simulink model "AvionicStateFlow1"  (R2021a)
settings: Solver=FixedStepAuto  StartTime=0.0  StopTime=inf  FixedStep=0.01  RelTol=1e-3  EnableMultiTasking=on
libraries: bbblueCommlib x27, svdutilitieslib x10, simulink x5, bbblueBasicLib x4, bbblueSensorLib x2
settings Model: SimulationMode=external  ExtModeTrigDuration=100  Creator=SONG PC  LastModifiedBy=sokserey
settings SolverCC: PositivePriorityOrder=on  AutoInsertRateTranBlk=on
settings OptimizationCC: EnhancedBackFolding=on  PassReuseOutputArgsAs=Individual arguments  ZeroExternalMemoryAtStartup=off  ZeroInternalMemoryAtStartup=off  MaxStackSize=64  OptimizeBlockOrder=speed  DifferentSizesBufferReuse=on  OptimizationCustomize=off  EfficientTunableParamExpr=on
settings DebuggingCC: ParameterTunabilityLossMsg=error
settings HardwareCC: ProdBitPerPointer=32  ProdBitPerSizeT=32  ProdBitPerPtrDiffT=32  ProdLargestAtomicInteger=Long  ProdLargestAtomicFloat=Double  ProdWordSize=32  ProdHWDeviceType=ARM Compatible->ARM Cortex
settings SFSimCC: MATLABDynamicMemAlloc=off
settings RTWCC: SystemTargetFile=ert.tlc  HardwareBoard=BeagleBone Blue  TLCOptions="-aInlineSetEventsForThisBaseRateFcn=TLC_FALSE -aSuppressMultiTaskScheduler=TLC_FALSE  -aRateBasedStepFcn=0"  TemplateMakefile=ert_default_tmf  Toolchain=GNU GCC BeagleBone Blue
settings CodeAppCC: ForceParamTrailComments=on  IgnoreCustomStorageClasses=off  OperatorAnnotations=on  SimulinkDataObjDesc=on  SFDataObjDesc=on  InsertBlockDesc=on
settings ERTTargetCC: SupportContinuousTime=on  SupportVariableSizeSignals=on  ExtMode=on  ExtModeMexArgs='192.168.7.2' 0 17725

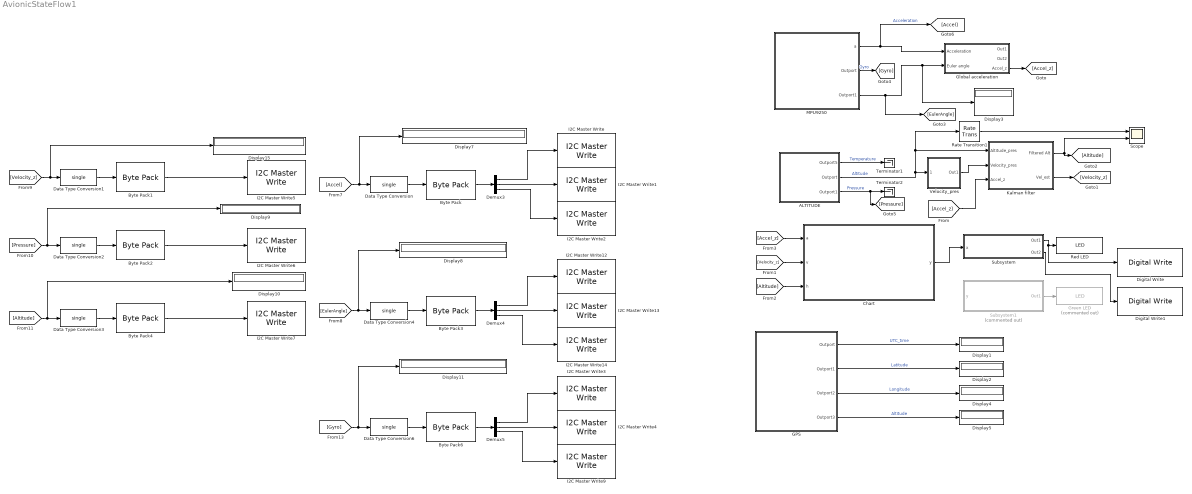
== system AvionicStateFlow1 ==
  "ALTITUDE " : Subsystem
  Byte Pack{,1..4,6} (6 alike) : svdutilitieslib/Byte Pack  maskPackedDataType=uint8  datatypes={'single'}  byteAlign=1  blockPlatform=arduinoert
      settings: SourceProductBaseCode=ARDUINO,ML_ARDUINO,ECCORTEXA,ECCORTEXR,SC_BEAGLEBONE_BLUE,EC_FREEDOM_BOARD,EC_FRDM_K64F,INTEL_BLOCKSET,MICROBIT,NUCLEO,PX4AUTOPILOTS,RASPPIIO,STMICRODIS,TIC2000,XILINX_BLOCKSET
  Chart : Stateflow chart  TreatAsAtomicUnit=on
  Data Type Conversion{,1..4,6} (6 alike) : DataTypeConversion  OutDataTypeStr=single
  Demux3 : Demux  Outputs=3
  Demux4 : Demux  Outputs=3
  Demux5 : Demux  Outputs=3
  Digital Write : bbblueBasicLib/Digital Write  GPIOSelect=GPIO1_25  Pin=49  Direction=output
      settings: SourceProductBaseCode=SC_BEAGLEBONE_BLUE
  Digital Write1 : bbblueBasicLib/Digital Write  GPIOSelect=GPIO3_2  Pin=49  Direction=output
      settings: SourceProductBaseCode=SC_BEAGLEBONE_BLUE
  Display{1..5,7..11,15} (11 alike) : Display
  GPS : Subsystem
  Global acceleration : Subsystem
  Green LED : bbblueBasicLib/LED  Commented=on  LED=Green
      settings: SourceProductBaseCode=SC_BEAGLEBONE_BLUE
  I2C Master Write{,1..7,9,12..14} (12 alike) : bbblueCommlib/I2C Master Write  I2CModule=1  Mode=Master  SlaveAddress=8  SlaveByteOrder=BigEndian  Direction=Transmitter  RegisterAddressMode=off  RegisterAddress=0  SlaveDataType=uint8  DataLength=1  NoAck=off  RepeatedStart=off  OutputStatus=off
      settings: SourceProductBaseCode=SC_BEAGLEBONE_BLUE
  Kalman filter : Subsystem
  MPU9250 : Subsystem
  Rate Transition1 : RateTransition
  Red LED : bbblueBasicLib/LED  LED=Red
      settings: SourceProductBaseCode=SC_BEAGLEBONE_BLUE
  Scope : Scope  NumInputPorts=2
  Subsystem : Subsystem
  Subsystem1 : Subsystem  Commented=on
  Terminator1 : Terminator
  Terminator2 : Terminator
  Velocity_pres : Subsystem
  wires:
  "ALTITUDE "/2(Outport) -> Velocity_pres/1(Altitude), Rate Transition1/1, Kalman filter/1(Altitude_pres)  "Altitude"
  "ALTITUDE "/3(Outport1) -> [Pressure], Terminator2/1  "Pressure"
  "ALTITUDE "/1(Outport5) -> Terminator1/1  "Temperature"
  Rate Transition1/1 -> Scope/1
  Subsystem/1(Out1) -> Digital Write/1, Red LED/1
  Subsystem1/1(Out1) -> Green LED/1
  MPU9250/1(a) -> [Accel], Global acceleration/1(Acceleration)  "Acceleration"
  Kalman filter/1(Filtered Alt) -> Scope/2, [Altitude]
  Kalman filter/2(Vel_est) -> [Velocity_z]
  Global acceleration/3(Accel_z) -> [Accel_z]
  [Accel_z] -> Kalman filter/3(Accel_z)
  [Accel_z] -> Chart/1(a)
  [Velocity_z] -> Chart/2(v)
  [Altitude] -> Chart/3(h)
  Velocity_pres/1(Out1) -> Kalman filter/2(Velocity_pres)
  Chart/1(y) -> Subsystem/1(x)
  Subsystem/2(Out2) -> Digital Write1/1
  Data Type Conversion6/1 -> Byte Pack6/1
  Byte Pack3/1 -> Demux4/1
  Demux5/1 -> I2C Master Write3/1
  Demux3/1 -> I2C Master Write/1
  Byte Pack2/1 -> I2C Master Write6/1
  [EulerAngle] -> Display8/1, Data Type Conversion4/1
  Byte Pack1/1 -> I2C Master Write5/1
  Data Type Conversion1/1 -> Byte Pack1/1
  Byte Pack6/1 -> Demux5/1
  Demux3/2 -> I2C Master Write1/1
  Byte Pack/1 -> Demux3/1
  Demux5/3 -> I2C Master Write9/1
  Demux4/3 -> I2C Master Write14/1
  Byte Pack4/1 -> I2C Master Write7/1
  [Altitude] -> Display10/1, Data Type Conversion3/1
  [Velocity_z] -> Display15/1, Data Type Conversion1/1
  Demux4/2 -> I2C Master Write13/1
  [Gyro] -> Display11/1, Data Type Conversion6/1
  Demux5/2 -> I2C Master Write4/1
  [Pressure] -> Display9/1, Data Type Conversion2/1
  [Accel] -> Display7/1, Data Type Conversion/1
  Demux4/1 -> I2C Master Write12/1
  Data Type Conversion3/1 -> Byte Pack4/1
  Data Type Conversion/1 -> Byte Pack/1
  Demux3/3 -> I2C Master Write2/1
  Data Type Conversion4/1 -> Byte Pack3/1
  Data Type Conversion2/1 -> Byte Pack2/1
  MPU9250/3(Outport1) -> [EulerAngle], Display3/1, Global acceleration/2(Euler angle)
  MPU9250/2(Outport) -> [Gyro]  "Gyro"
  GPS/2(Outport1) -> Display2/1  "Latitude"
  GPS/3(Outport2) -> Display4/1  "Longitude"
  GPS/4(Outport3) -> Display5/1  "Altitude"
  GPS/1(Outport) -> Display1/1  "UTC_time"

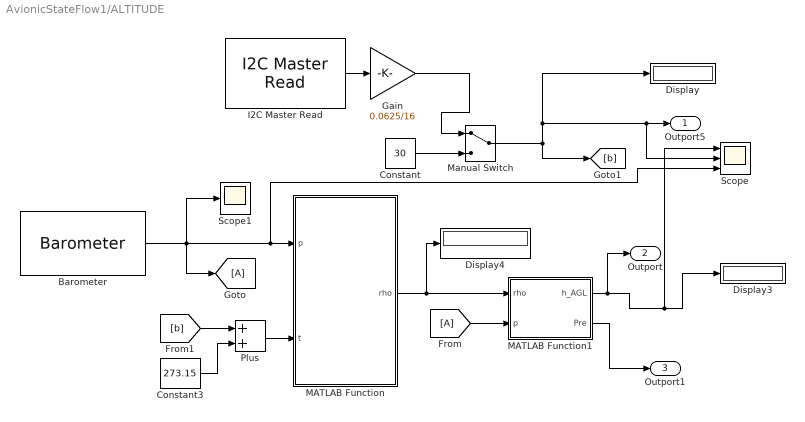
== system AvionicStateFlow1/ALTITUDE  ==
  Barometer : bbblueSensorLib/Barometer  OSRSelection=16  IIRFilterCoeff=16  SampleTime=0.01
      settings: SourceProductBaseCode=SC_BEAGLEBONE_BLUE
  Constant : Constant  Value=30
  Constant3 : Constant  Value=273.15
  Display : Display
  Display3 : Display
  Display4 : Display
  Gain : Gain  Gain=0.0625/16  OutDataTypeStr=single
  I2C Master Read : bbblueCommlib/I2C Master Read  I2CModule=1  Mode=Master  SlaveAddress=hex2dec('48')  SlaveByteOrder=BigEndian  Direction=Receiver  RegisterAddressMode=off  RegisterAddress=0  SlaveDataType=int16  DataLength=1  NoAck=off  RepeatedStart=off  OutputStatus=off  SampleTime=0.01
      settings: SourceProductBaseCode=SC_BEAGLEBONE_BLUE
  MATLAB Function : MATLAB Function  TreatAsAtomicUnit=on
  MATLAB Function1 : MATLAB Function  TreatAsAtomicUnit=on
  Manual Switch : ManualSwitch
  Plus : Sum
  Scope : Scope  NumInputPorts=3
  Scope1 : Scope
  Outport5 : Outport
  Outport : Outport  Port=2
  Outport1 : Outport  Port=3
  wires:
  I2C Master Read/1 -> Gain/1
  Plus/1 -> MATLAB Function/2(t)
  Barometer/1 -> Scope1/1, [A], Scope/3, MATLAB Function/1(p)
  Gain/1 -> Manual Switch/1
  MATLAB Function/1(rho) -> Display4/1, MATLAB Function1/1(rho)
  Constant3/1 -> Plus/2
  [A] -> MATLAB Function1/2(p)
  [b] -> Plus/1
  MATLAB Function1/1(h_AGL) -> Outport/1, Display3/1, Scope/1
  MATLAB Function1/2(Pre) -> Outport1/1
  Constant/1 -> Manual Switch/2
  Manual Switch/1 -> [b], Display/1, Scope/2, Outport5/1

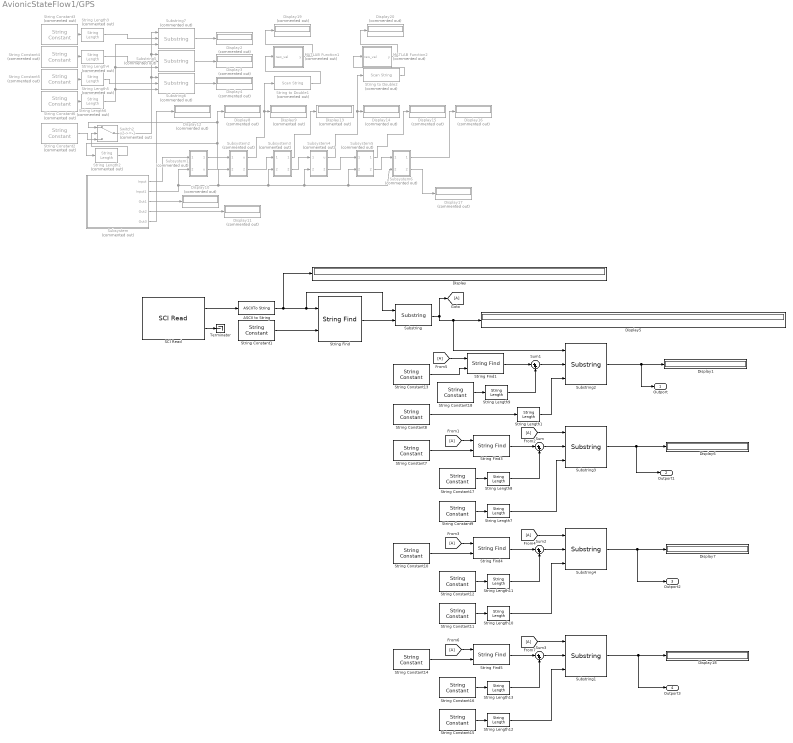
== system AvionicStateFlow1/GPS ==
  ASCII to String : ASCIIToString
  Display{,1,5..7,18} (6 alike) : Display
  Display{2..4,8..17,19..20} (15 alike) : Display  Commented=on
  MATLAB Function1 : MATLAB Function  Commented=on  TreatAsAtomicUnit=on
  MATLAB Function2 : MATLAB Function  Commented=on  TreatAsAtomicUnit=on
  SCI Read : bbblueCommlib/SCI Read  SCIModule=/dev/ttyO2  BaudrateOptions=9600  Parity=None  StopbitOptions=1  Baudrate=uint32(9600)  StopBits=1  HardwareFlowControl=None  ByteOrder=LittleEndian  DataType=uint8  DataLength=150  OutputStatus=on  SampleTime=0.1
      settings: SourceProductBaseCode=SC_BEAGLEBONE_BLUE
  String Constant1 : StringConstant  String="\"$GPGGA\""
  String Constant{7,10,13..14} (4 alike) : StringConstant  String="\",\""
  String Constant11 : StringConstant  String="\"hhhhhhhhhh\""
  String Constant12 : StringConstant  String="\"123456789101111111111111\""
  String Constant15 : StringConstant  String="\"hhhh\""
  String Constant16 : StringConstant  String="\"123456789101111111111111111111111111111111111111\""
  String Constant17 : StringConstant  String="\"12345678910\""
  String Constant18 : StringConstant  String="\"1\""
  String Constant2 : StringConstant  Commented=on  String="\"000000\""
  String Constant3 : StringConstant  Commented=on  String="\"0\""
  String Constant4 : StringConstant  Commented=on  String="\"000\""
  String Constant5 : StringConstant  Commented=on  String="\"00000\""
  String Constant6 : StringConstant  Commented=on  String="\"00\""
  String Constant8 : StringConstant  String="\"hhhhhh\""
  String Constant9 : StringConstant  String="\"hhhhhhhhhh\""
  String Find{,1,3..5} (5 alike) : StringFind
  String Length{1,7,10,12} (4 alike) : StringLength
  String Length{8..9,11,13} (4 alike) : StringLength  OutDataTypeStr=int32
  String Length{2..6} (5 alike) : StringLength  Commented=on
  String to Double1 : ScanString  Commented=on  Format="\"%lf\""
  String to Double2 : ScanString  Commented=on  Format="\"%lf\""
  Substring : Substring  StringFromIdxToEnd=on
  Substring{1..4} (4 alike) : Substring
  Substring5 : Substring  Commented=on
  Substring6 : Substring  Commented=on
  Substring7 : Substring  Commented=on
  Subsystem : Subsystem  Commented=on
  Subsystem1 : Subsystem  Commented=on
  Subsystem2 : Subsystem  Commented=on
  Subsystem3 : Subsystem  Commented=on
  Subsystem4 : Subsystem  Commented=on
  Subsystem5 : Subsystem  Commented=on
  Subsystem6 : Subsystem  Commented=on
  Sum{,1..3} (4 alike) : Sum  Inputs=|++
  Switch2 : Switch  Commented=on  Threshold=1
  Terminator : Terminator
  Outport : Outport
  Outport1 : Outport  Port=2
  Outport2 : Outport  Port=3
  Outport3 : Outport  Port=4
  wires:
  Switch2/1 -> Substring6/1, Substring5/1, Substring7/1
  String Length6/1 -> Substring6/3, Substring7/3, Substring5/3
  String Length4/1 -> Substring5/2
  String Length3/1 -> Substring7/2
  Subsystem5/1(Out1) -> Display15/1
  Subsystem/5(Out3) -> Display12/1
  Substring6/1 -> Display4/1
  String Constant5/1 -> String Length5/1
  String Constant4/1 -> String Length4/1
  String Length2/1 -> Switch2/2
  String Constant2/1 -> Switch2/3
  String Constant3/1 -> String Length3/1
  MATLAB Function2/1(y) -> Display20/1
  String to Double2/1 -> MATLAB Function2/1(raw_val)
  Subsystem6/2(Out2) -> Display17/1
  Subsystem3/1(Out1) -> Display13/1
  Subsystem3/2(Out2) -> Subsystem4/1(In1)
  Subsystem2/1(u) -> String to Double1/1, Display9/1
  Subsystem4/1(u) -> String to Double2/1, Display14/1
  Subsystem5/2(Out2) -> Subsystem6/1(In1)
  Subsystem4/2(Out2) -> Subsystem5/1(In1)
  String Length5/1 -> Substring6/2
  Subsystem/4(Out2) -> Display11/1
  String Constant6/1 -> String Length6/1
  MATLAB Function1/1(y) -> Display19/1
  Subsystem1/1(Out1) -> Subsystem2/1(In1)
  String to Double1/1 -> MATLAB Function1/1(raw_val)
  Subsystem/1(Input) -> Subsystem1/1(Input)
  Subsystem6/1(Out1) -> Display16/1
  Subsystem/3(Out1) -> Display10/1
  Subsystem/2(Input1) -> Subsystem1/2(Input1), Subsystem6/2(Input1), Subsystem5/2(Input1), Subsystem4/2(Input1), Subsystem3/2(Input1), Subsystem2/2(Input1)
  Subsystem2/2(Out2) -> Subsystem3/1(In1)
  Subsystem1/2(u) -> String Length2/1, Switch2/1, Display8/1
  Substring5/1 -> Display3/1
  Substring7/1 -> Display2/1
  [A] -> String Find3/1
  String Constant9/1 -> String Length7/1
  String Length7/1 -> Substring3/3
  Substring3/1 -> Outport1/1, Display6/1
  Substring1/1 -> Outport3/1, Display18/1
  String Constant16/1 -> String Length13/1
  [A] -> Substring1/1
  String Constant18/1 -> String Length9/1
  String Find5/1 -> Sum3/1
  [A] -> String Find5/1
  [A] -> Substring3/1
  String Find4/1 -> Sum2/1
  String Length10/1 -> Substring4/3
  String Find3/1 -> Sum/1
  String Length12/1 -> Substring1/3
  String Constant10/1 -> String Find4/2
  String Length11/1 -> Sum2/2
  [A] -> String Find4/1
  String Constant11/1 -> String Length10/1
  [A] -> Substring4/1
  String Constant12/1 -> String Length11/1
  String Constant13/1 -> String Find1/2
  [A] -> String Find1/1
  Sum2/1 -> Substring4/2
  String Length9/1 -> Sum1/2
  String Find1/1 -> Sum1/1
  String Length8/1 -> Sum/2
  String Length1/1 -> Substring2/3
  String Constant1/1 -> String Find/2
  Substring2/1 -> Outport/1, Display1/1
  String Constant15/1 -> String Length12/1
  Sum1/1 -> Substring2/2
  String Constant8/1 -> String Length1/1
  SCI Read/1 -> ASCII to String/1
  String Constant7/1 -> String Find3/2
  ASCII to String/1 -> Substring/1, String Find/1, Display/1
  Substring4/1 -> Outport2/1, Display7/1
  String Find/1 -> Substring/2
  Sum3/1 -> Substring1/2
  Substring/1 -> Substring2/1, Display5/1, [A]
  Sum/1 -> Substring3/2
  String Length13/1 -> Sum3/2
  String Constant14/1 -> String Find5/2
  String Constant17/1 -> String Length8/1
  SCI Read/2 -> Terminator/1

== system AvionicStateFlow1/Global acceleration ==
  Acceleration : Inport
  Euler angle : Inport  Port=2
  Demux : Demux  Outputs=3
  Display : Display
  Display1 : Display
  MATLAB Function : MATLAB Function  TreatAsAtomicUnit=on
  Out1 : Outport
  Out2 : Outport  Port=2
  Accel_z : Outport  Port=3
  wires:
  Acceleration/1 -> MATLAB Function/1(a), Display1/1
  MATLAB Function/1(acc) -> Display/1, Demux/1
  Demux/1 -> Out1/1
  Demux/3 -> Accel_z/1
  Euler angle/1 -> MATLAB Function/2(b)
  Demux/2 -> Out2/1

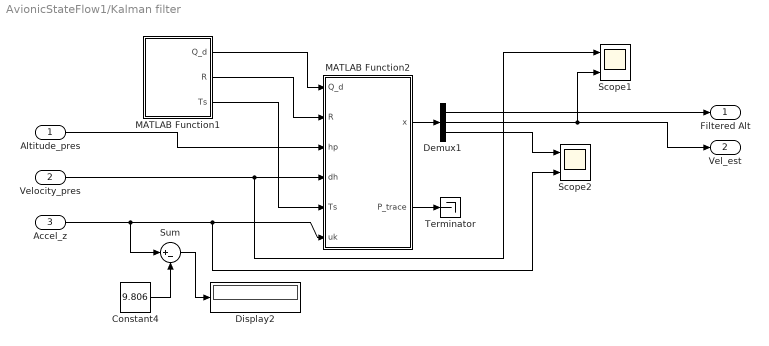
== system AvionicStateFlow1/Kalman filter ==
  Altitude_pres : Inport
  Velocity_pres : Inport  Port=2
  Accel_z : Inport  Port=3
  Constant4 : Constant  Value=9.806
  Demux1 : Demux  Outputs=3
  Display2 : Display
  MATLAB Function1 : MATLAB Function  TreatAsAtomicUnit=on
  MATLAB Function2 : MATLAB Function  TreatAsAtomicUnit=on
  Scope1 : Scope  NumInputPorts=2
  Scope2 : Scope  NumInputPorts=2
  Sum : Sum  Inputs=|+-
  Terminator : Terminator
  Filtered Alt : Outport
  Vel_est : Outport  Port=2
  wires:
  Demux1/2 -> Vel_est/1, Scope1/2
  MATLAB Function1/3(Ts) -> MATLAB Function2/5(Ts)
  Velocity_pres/1 -> MATLAB Function2/4(dh), Scope1/1
  Constant4/1 -> Sum/2
  MATLAB Function2/1(x) -> Demux1/1
  Demux1/3 -> Scope2/1
  MATLAB Function1/2(R) -> MATLAB Function2/2(R)
  Sum/1 -> Display2/1
  MATLAB Function2/2(P_trace) -> Terminator/1
  Altitude_pres/1 -> MATLAB Function2/3(hp)
  MATLAB Function1/1(Q_d) -> MATLAB Function2/1(Q_d)
  Accel_z/1 -> Scope2/2, MATLAB Function2/6(uk), Sum/1
  Demux1/1 -> Filtered Alt/1

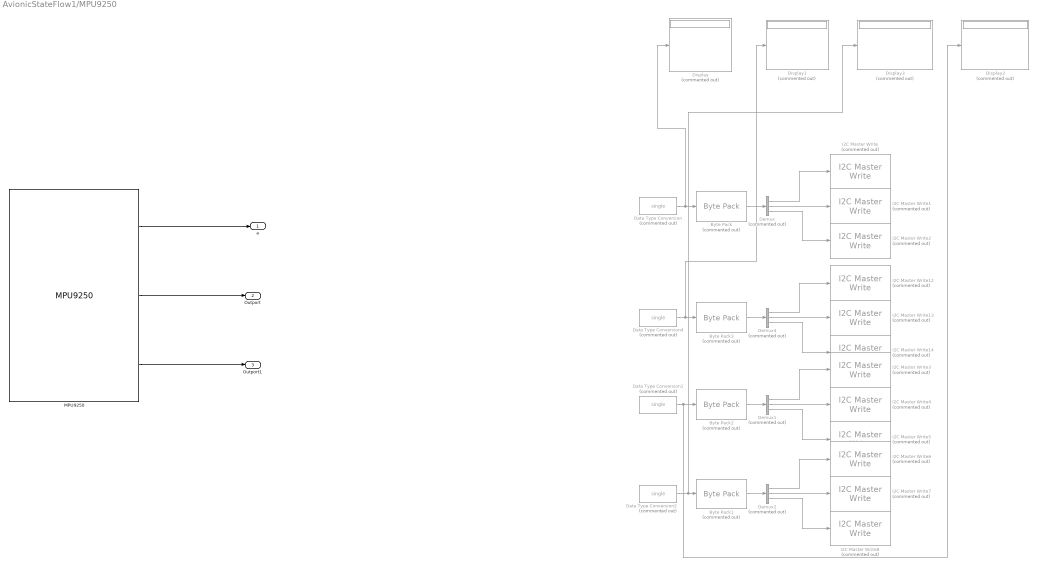
== system AvionicStateFlow1/MPU9250 ==
  Byte Pack{,1..3} (4 alike) : svdutilitieslib/Byte Pack  Commented=on  maskPackedDataType=uint8  datatypes={'single'}  byteAlign=1  blockPlatform=arduinoert
      settings: SourceProductBaseCode=ANDROID,ARDUINO,ML_ARDUINO,ECCORTEXA,ECCORTEXR,SC_BEAGLEBONE_BLUE,EC_FREEDOM_BOARD,EC_FRDM_K64F,INTEL_BLOCKSET,MICROBIT,NUCLEO,NVIDIA,PX4AUTOPILOTS,RASPPIIO,STMICRODIS,TIC2000,XILINX_BLOCKSET
  Data Type Conversion{,1..2,4} (4 alike) : DataTypeConversion  Commented=on  OutDataTypeStr=single
  Demux{,1..2,4} (4 alike) : Demux  Commented=on  Outputs=3
  Display{,1..3} (4 alike) : Display  Commented=on
  I2C Master Write{,1..8,12..14} (12 alike) : bbblueCommlib/I2C Master Write  Commented=on  I2CModule=1  Mode=Master  SlaveAddress=8  SlaveByteOrder=BigEndian  Direction=Transmitter  RegisterAddressMode=off  RegisterAddress=0  SlaveDataType=uint8  DataLength=1  NoAck=off  RepeatedStart=off  OutputStatus=off
      settings: SourceProductBaseCode=SC_BEAGLEBONE_BLUE
  MPU9250 : bbblueSensorLib/MPU9250  OperationMode=DMP  Accel=on  AngularRate=on  Ak8963Field=off  EulerAngles=on  Quat=off  AccelRange=16G  Acceldlpf=1  GyroRange=250 dps  Gyrodlpf=1  DmpOdr=200 Hz  SampleTime=0.01
      settings: SourceProductBaseCode=SC_BEAGLEBONE_BLUE
  a : Outport
  Outport : Outport  Port=2
  Outport1 : Outport  Port=3
  wires:
  MPU9250/1 -> a/1
  Demux/1 -> I2C Master Write/1
  Demux/2 -> I2C Master Write1/1
  Byte Pack/1 -> Demux/1
  Demux/3 -> I2C Master Write2/1
  MPU9250/2 -> Outport/1
  Data Type Conversion/1 -> Display/1, Byte Pack/1
  Demux4/1 -> I2C Master Write12/1
  Byte Pack3/1 -> Demux4/1
  Data Type Conversion4/1 -> Byte Pack3/1, Display1/1
  Demux4/2 -> I2C Master Write13/1
  Demux4/3 -> I2C Master Write14/1
  Demux1/3 -> I2C Master Write5/1
  Data Type Conversion1/1 -> Byte Pack2/1, Display2/1
  Byte Pack2/1 -> Demux1/1
  Demux1/1 -> I2C Master Write3/1
  Demux1/2 -> I2C Master Write4/1
  Demux2/3 -> I2C Master Write8/1
  Data Type Conversion2/1 -> Byte Pack1/1, Display3/1
  Byte Pack1/1 -> Demux2/1
  Demux2/1 -> I2C Master Write6/1
  Demux2/2 -> I2C Master Write7/1
  MPU9250/3 -> Outport1/1

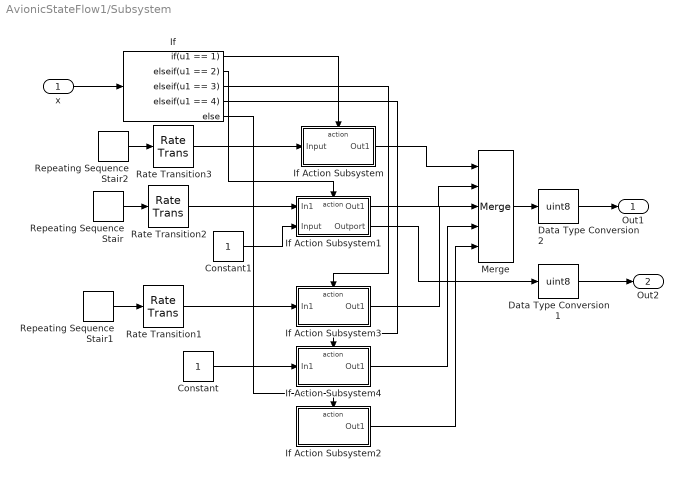
== system AvionicStateFlow1/Subsystem ==
  x : Inport
  Constant : Constant
  Constant1 : Constant
  Data Type Conversion1 : DataTypeConversion  OutDataTypeStr=uint8
  Data Type Conversion2 : DataTypeConversion  OutDataTypeStr=uint8
  If : If  IfExpression=u1 == 1  ElseIfExpressions=u1 == 2, u1 == 3, u1 == 4
  If Action Subsystem : Subsystem  TreatAsAtomicUnit=on
  If Action Subsystem1 : Subsystem  TreatAsAtomicUnit=on
  If Action Subsystem2 : Subsystem  TreatAsAtomicUnit=on
  If Action Subsystem3 : Subsystem  TreatAsAtomicUnit=on
  If Action Subsystem4 : Subsystem  TreatAsAtomicUnit=on
  Merge : Merge  Inputs=5
  Rate Transition1 : RateTransition
  Rate Transition2 : RateTransition
  Rate Transition3 : RateTransition
  Repeating Sequence Stair : simulink/Sources/Repeating Sequence Stair  OutValues=[1 0 1 0 1 0 0 0].'  tsamp=0.1  OutMin=[]  OutMax=[]  OutDataTypeStr=double  OutputDataTypeScalingMode=double  OutDataType=fixdt(0,8)  ConRadixGroup=Best Precision: Vector-wise  OutScaling=2^-12
  Repeating Sequence Stair1 : simulink/Sources/Repeating Sequence Stair  OutValues=[1 0 1 0 0 0 0 0].'  tsamp=0.1  OutMin=[]  OutMax=[]  OutDataTypeStr=double  OutputDataTypeScalingMode=double  OutDataType=fixdt(0,8)  ConRadixGroup=Best Precision: Vector-wise  OutScaling=2^-12
  Repeating Sequence Stair2 : simulink/Sources/Repeating Sequence Stair  OutValues=[1 1 1 1 1 0 0 0 0 0].'  tsamp=0.1  OutMin=[]  OutMax=[]  OutDataTypeStr=double  OutputDataTypeScalingMode=double  OutDataType=fixdt(0,8)  ConRadixGroup=Best Precision: Vector-wise  OutScaling=2^-12
  Out1 : Outport
  Out2 : Outport  Port=2
  wires:
  If/5 -> If Action Subsystem2/Action
  If Action Subsystem2/1(Out1) -> Merge/5
  If/1 -> If Action Subsystem/Action
  Repeating Sequence Stair/1 -> Rate Transition2/1
  Rate Transition2/1 -> If Action Subsystem1/1(In1)
  Merge/1 -> Data Type Conversion2/1
  If Action Subsystem/1(Out1) -> Merge/1
  If Action Subsystem1/1(Out1) -> Merge/2
  If/2 -> If Action Subsystem1/Action
  Data Type Conversion2/1 -> Out1/1
  x/1 -> If/1
  Repeating Sequence Stair1/1 -> Rate Transition1/1
  Rate Transition1/1 -> If Action Subsystem3/1(In1)
  If/3 -> If Action Subsystem3/Action
  If Action Subsystem3/1(Out1) -> Merge/3
  If Action Subsystem4/1(Out1) -> Merge/4
  Constant/1 -> If Action Subsystem4/1(In1)
  If/4 -> If Action Subsystem4/Action
  Repeating Sequence Stair2/1 -> Rate Transition3/1
  Rate Transition3/1 -> If Action Subsystem/1(Input)
  Data Type Conversion1/1 -> Out2/1
  Constant1/1 -> If Action Subsystem1/2(Input)
  If Action Subsystem1/2(Outport) -> Data Type Conversion1/1

== system AvionicStateFlow1/Subsystem1 ==
  y : Inport
  Constant1 : Constant  Value=0
  Data Type Conversion1 : DataTypeConversion  OutDataTypeStr=uint8
  Rate Transition2 : RateTransition
  Repeating Sequence Stair : simulink/Sources/Repeating Sequence Stair  OutValues=[1 1 1 1 1 0 0 0 0 0].'  tsamp=0.1  OutMin=[]  OutMax=[]  OutDataTypeStr=double  OutputDataTypeScalingMode=double  OutDataType=fixdt(0,8)  ConRadixGroup=Best Precision: Vector-wise  OutScaling=2^-12
  Switch1 : Switch  Criteria=u2 > Threshold
  Out1 : Outport
  wires:
  Rate Transition2/1 -> Switch1/1
  Switch1/1 -> Data Type Conversion1/1
  Constant1/1 -> Switch1/3
  Data Type Conversion1/1 -> Out1/1
  y/1 -> Switch1/2
  Repeating Sequence Stair/1 -> Rate Transition2/1

== system AvionicStateFlow1/Velocity_pres ==
  Altitude : Inport
  Discrete Derivative : simulink/Discrete/Discrete Derivative  gainval=1.0  ICPrevScaledInput=0.0  OutMin=[]  OutMax=[]  OutDataType=fixdt(1, 16)  OutScaling=2^-10  DoSatur=off
  Rate Transition : RateTransition  OutPortSampleTime=0.2
  Rate Transition3 : RateTransition
  Out1 : Outport
  wires:
  Discrete Derivative/1 -> Rate Transition3/1
  Rate Transition/1 -> Discrete Derivative/1
  Rate Transition3/1 -> Out1/1
  Altitude/1 -> Rate Transition/1

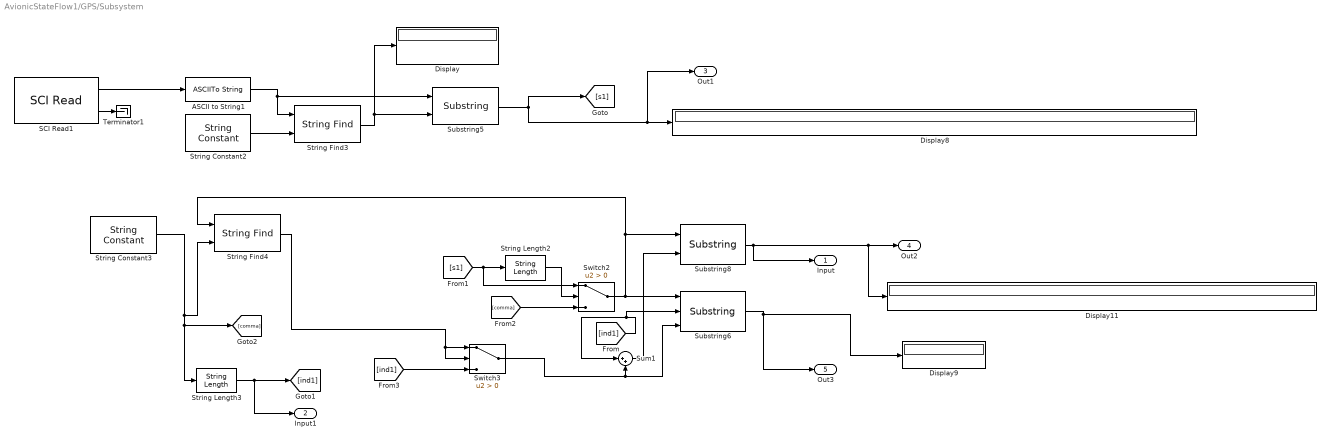
== system AvionicStateFlow1/GPS/Subsystem ==
  ASCII to String1 : ASCIIToString
  Display{,8..9,11} (4 alike) : Display
  SCI Read1 : bbblueCommlib/SCI Read  SCIModule=/dev/ttyO1  BaudrateOptions=9600  Parity=None  StopbitOptions=1  Baudrate=uint32(9600)  StopBits=1  HardwareFlowControl=None  ByteOrder=LittleEndian  DataType=uint8  DataLength=100  OutputStatus=on  SampleTime=0.1
      settings: SourceProductBaseCode=SC_BEAGLEBONE_BLUE
  String Constant2 : StringConstant  String="\"$GPGGA\""
  String Constant3 : StringConstant  String="\",\""
  String Find3 : StringFind
  String Find4 : StringFind
  String Length2 : StringLength
  String Length3 : StringLength
  Substring5 : Substring  InheritMaximumLength=off  StringFromIdxToEnd=on
  Substring6 : Substring
  Substring8 : Substring  StringFromIdxToEnd=on
  Sum1 : Sum  Inputs=|++
  Switch2 : Switch  Criteria=u2 > Threshold
  Switch3 : Switch  Criteria=u2 > Threshold
  Terminator1 : Terminator
  Input : Outport
  Input1 : Outport  Port=2
  Out1 : Outport  Port=3
  Out2 : Outport  Port=4
  Out3 : Outport  Port=5
  wires:
  Sum1/1 -> Substring8/2
  Substring6/1 -> Out3/1, Display9/1
  [s1] -> Switch2/1, String Length2/1
  Switch3/1 -> Substring6/3, Sum1/2
  String Constant2/1 -> String Find3/2
  [comma] -> Switch2/3
  ASCII to String1/1 -> Substring5/1, String Find3/1
  String Find4/1 -> Switch3/2, Switch3/1
  Switch2/1 -> Substring8/1, String Find4/1, Substring6/1
  String Constant3/1 -> String Find4/2, String Length3/1, [comma]
  SCI Read1/2 -> Terminator1/1
  String Find3/1 -> Substring5/2, Display/1
  SCI Read1/1 -> ASCII to String1/1
  String Length2/1 -> Switch2/2
  Substring8/1 -> Input/1, Display11/1, Out2/1
  [ind1] -> Switch3/3
  [ind1] -> Sum1/1, Substring6/2
  Substring5/1 -> Out1/1, Display8/1, [s1]
  String Length3/1 -> Input1/1, [ind1]

== system AvionicStateFlow1/GPS/Subsystem1 ==
  Input : Inport
  Input1 : Inport  Port=2
  String Constant : StringConstant  String="\",\""
  String Constant5 : StringConstant  String="\"1\""
  String Find5 : StringFind
  String Length4 : StringLength
  Substring7 : Substring
  Substring9 : Substring  StringFromIdxToEnd=on
  Sum2 : Sum  Inputs=|++
  Switch4 : Switch  Criteria=u2 > Threshold
  Switch5 : Switch  Criteria=u2 > Threshold
  Out1 : Outport
  u : Outport  Port=2
  wires:
  Sum2/1 -> Substring9/2
  String Constant5/1 -> Switch4/3
  Substring9/1 -> Out1/1
  String Find5/1 -> Switch5/2, Switch5/1
  Switch4/1 -> Substring9/1, String Find5/1, Substring7/1
  String Length4/1 -> Switch4/2
  Input/1 -> Switch4/1, String Length4/1
  String Constant/1 -> String Find5/2
  Switch5/1 -> Sum2/2, Substring7/3
  Input1/1 -> Switch5/3, Substring7/2, Sum2/1
  Substring7/1 -> u/1

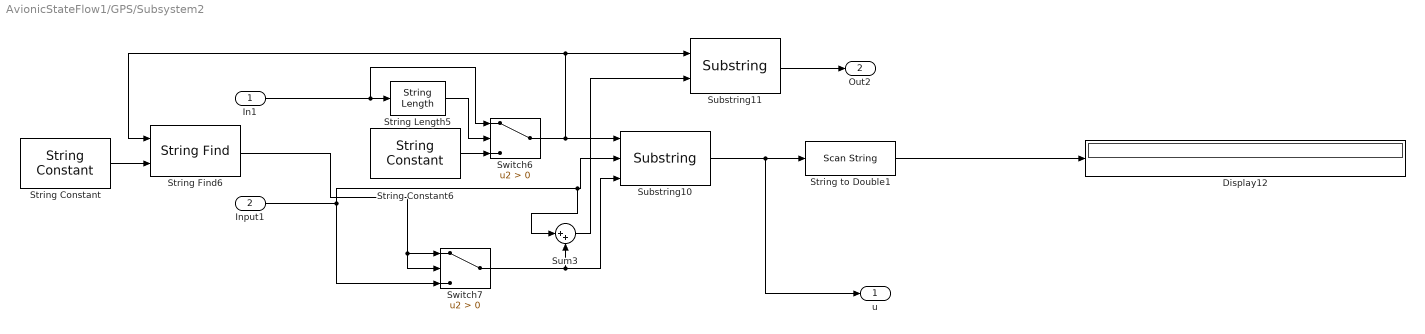
== system AvionicStateFlow1/GPS/Subsystem2 ==
  In1 : Inport
  Input1 : Inport  Port=2
  Display12 : Display
  String Constant : StringConstant  String="\",\""
  String Constant6 : StringConstant  String="\"1\""
  String Find6 : StringFind
  String Length5 : StringLength
  String to Double1 : ScanString  Format="\"%lf\""
  Substring10 : Substring
  Substring11 : Substring  StringFromIdxToEnd=on
  Sum3 : Sum  Inputs=|++
  Switch6 : Switch  Criteria=u2 > Threshold
  Switch7 : Switch  Criteria=u2 > Threshold
  u : Outport
  Out2 : Outport  Port=2
  wires:
  String Constant/1 -> String Find6/2
  String to Double1/1 -> Display12/1
  String Find6/1 -> Switch7/1, Switch7/2
  Switch6/1 -> Substring10/1, String Find6/1, Substring11/1
  Switch7/1 -> Substring10/3, Sum3/2
  String Length5/1 -> Switch6/2
  Substring10/1 -> u/1, String to Double1/1
  String Constant6/1 -> Switch6/3
  In1/1 -> String Length5/1, Switch6/1
  Input1/1 -> Switch7/3, Substring10/2, Sum3/1
  Substring11/1 -> Out2/1
  Sum3/1 -> Substring11/2

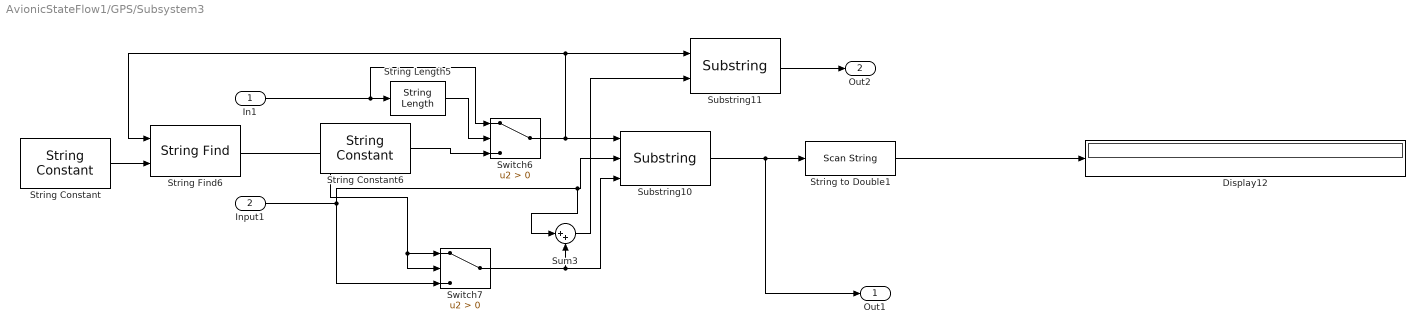
== system AvionicStateFlow1/GPS/Subsystem3 ==
  In1 : Inport
  Input1 : Inport  Port=2
  Display12 : Display
  String Constant : StringConstant  String="\",\""
  String Constant6 : StringConstant  String="\"1\""
  String Find6 : StringFind
  String Length5 : StringLength
  String to Double1 : ScanString  Format="\"%lf\""
  Substring10 : Substring
  Substring11 : Substring  StringFromIdxToEnd=on
  Sum3 : Sum  Inputs=|++
  Switch6 : Switch  Criteria=u2 > Threshold
  Switch7 : Switch  Criteria=u2 > Threshold
  Out1 : Outport
  Out2 : Outport  Port=2
  wires:
  Sum3/1 -> Substring11/2
  Substring11/1 -> Out2/1
  Input1/1 -> Sum3/1, Substring10/2, Switch7/3
  In1/1 -> Switch6/1, String Length5/1
  String Constant6/1 -> Switch6/3
  Substring10/1 -> String to Double1/1, Out1/1
  String Length5/1 -> Switch6/2
  Switch7/1 -> Sum3/2, Substring10/3
  Switch6/1 -> Substring11/1, String Find6/1, Substring10/1
  String Find6/1 -> Switch7/2, Switch7/1
  String to Double1/1 -> Display12/1
  String Constant/1 -> String Find6/2

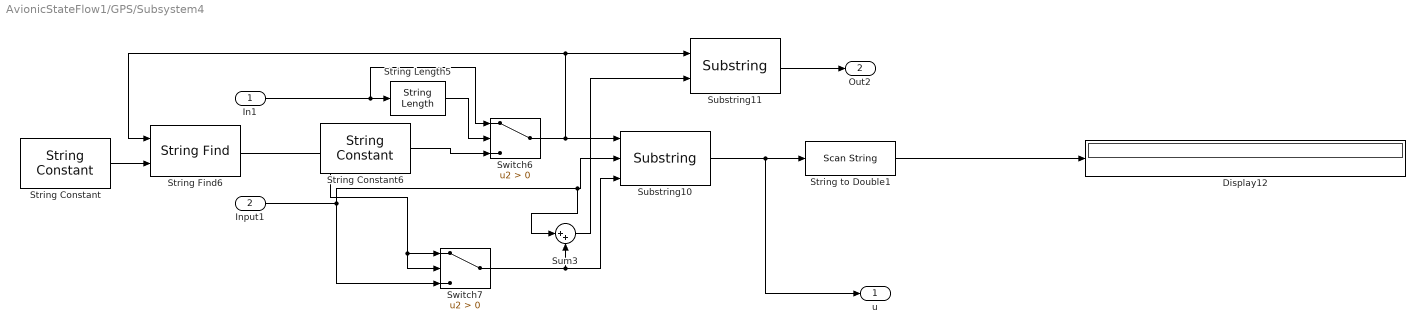
== system AvionicStateFlow1/GPS/Subsystem4 ==
  In1 : Inport
  Input1 : Inport  Port=2
  Display12 : Display
  String Constant : StringConstant  String="\",\""
  String Constant6 : StringConstant  String="\"1\""
  String Find6 : StringFind
  String Length5 : StringLength
  String to Double1 : ScanString  Format="\"%lf\""
  Substring10 : Substring
  Substring11 : Substring  StringFromIdxToEnd=on
  Sum3 : Sum  Inputs=|++
  Switch6 : Switch  Criteria=u2 > Threshold
  Switch7 : Switch  Criteria=u2 > Threshold
  u : Outport
  Out2 : Outport  Port=2
  wires:
  String Constant/1 -> String Find6/2
  String to Double1/1 -> Display12/1
  String Find6/1 -> Switch7/1, Switch7/2
  Switch6/1 -> Substring10/1, String Find6/1, Substring11/1
  Switch7/1 -> Substring10/3, Sum3/2
  String Length5/1 -> Switch6/2
  Substring10/1 -> u/1, String to Double1/1
  String Constant6/1 -> Switch6/3
  In1/1 -> String Length5/1, Switch6/1
  Input1/1 -> Switch7/3, Substring10/2, Sum3/1
  Substring11/1 -> Out2/1
  Sum3/1 -> Substring11/2

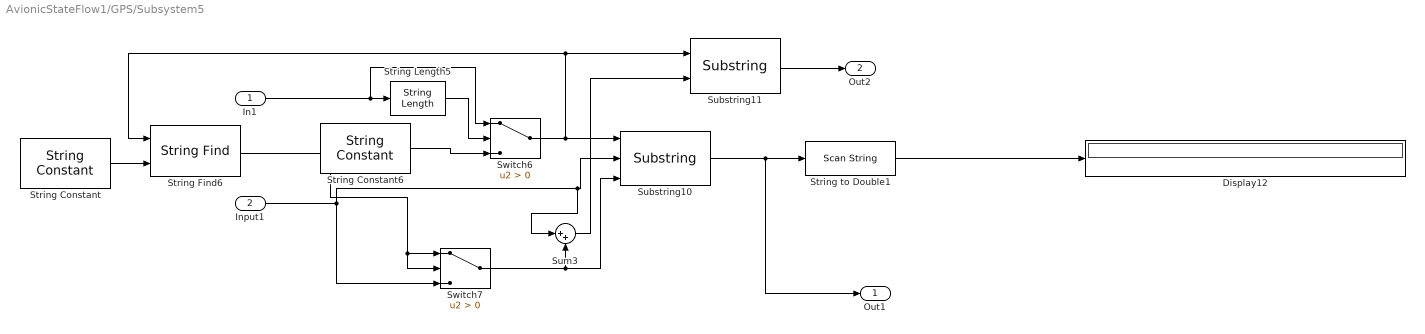
== system AvionicStateFlow1/GPS/Subsystem5 ==
  In1 : Inport
  Input1 : Inport  Port=2
  Display12 : Display
  String Constant : StringConstant  String="\",\""
  String Constant6 : StringConstant  String="\"1\""
  String Find6 : StringFind
  String Length5 : StringLength
  String to Double1 : ScanString  Format="\"%lf\""
  Substring10 : Substring
  Substring11 : Substring  StringFromIdxToEnd=on
  Sum3 : Sum  Inputs=|++
  Switch6 : Switch  Criteria=u2 > Threshold
  Switch7 : Switch  Criteria=u2 > Threshold
  Out1 : Outport
  Out2 : Outport  Port=2
  wires:
  String Constant/1 -> String Find6/2
  String to Double1/1 -> Display12/1
  String Find6/1 -> Switch7/1, Switch7/2
  Switch6/1 -> Substring10/1, String Find6/1, Substring11/1
  Switch7/1 -> Substring10/3, Sum3/2
  String Length5/1 -> Switch6/2
  Substring10/1 -> Out1/1, String to Double1/1
  String Constant6/1 -> Switch6/3
  In1/1 -> String Length5/1, Switch6/1
  Input1/1 -> Switch7/3, Substring10/2, Sum3/1
  Substring11/1 -> Out2/1
  Sum3/1 -> Substring11/2

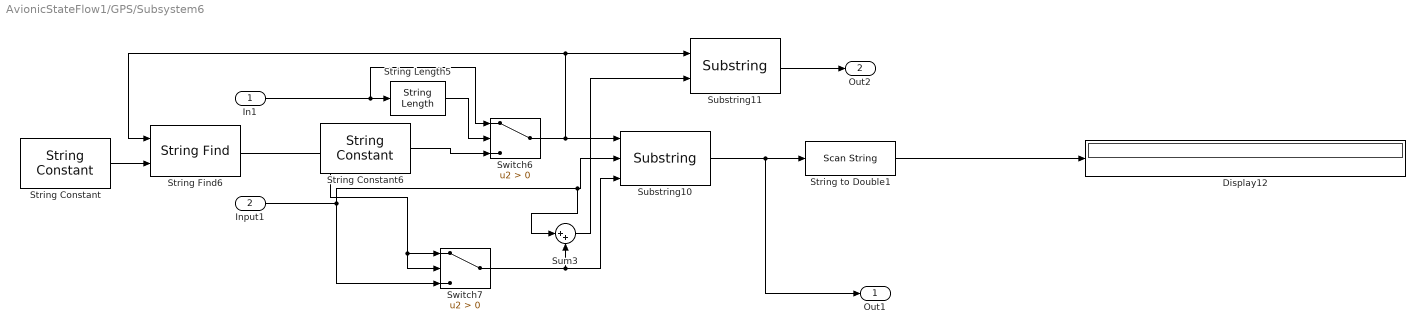
== system AvionicStateFlow1/GPS/Subsystem6 ==
  In1 : Inport
  Input1 : Inport  Port=2
  Display12 : Display
  String Constant : StringConstant  String="\",\""
  String Constant6 : StringConstant  String="\"1\""
  String Find6 : StringFind
  String Length5 : StringLength
  String to Double1 : ScanString  Format="\"%lf\""
  Substring10 : Substring
  Substring11 : Substring  StringFromIdxToEnd=on
  Sum3 : Sum  Inputs=|++
  Switch6 : Switch  Criteria=u2 > Threshold
  Switch7 : Switch  Criteria=u2 > Threshold
  Out1 : Outport
  Out2 : Outport  Port=2
  wires:
  Sum3/1 -> Substring11/2
  Substring11/1 -> Out2/1
  Input1/1 -> Sum3/1, Substring10/2, Switch7/3
  In1/1 -> Switch6/1, String Length5/1
  String Constant6/1 -> Switch6/3
  Substring10/1 -> String to Double1/1, Out1/1
  String Length5/1 -> Switch6/2
  Switch7/1 -> Sum3/2, Substring10/3
  Switch6/1 -> Substring11/1, String Find6/1, Substring10/1
  String Find6/1 -> Switch7/2, Switch7/1
  String to Double1/1 -> Display12/1
  String Constant/1 -> String Find6/2

== system AvionicStateFlow1/Subsystem/If Action Subsystem ==
  Input : Inport
  Action Port : ActionPort  ActionPortLabel=if(u1 == 1)
  Out1 : Outport
  wires:
  Input/1 -> Out1/1

== system AvionicStateFlow1/Subsystem/If Action Subsystem1 ==
  In1 : Inport
  Input : Inport  Port=2
  Action Port : ActionPort  ActionPortLabel=elseif(u1 == 2)
  Out1 : Outport
  Outport : Outport  Port=2
  wires:
  In1/1 -> Out1/1
  Input/1 -> Outport/1

== system AvionicStateFlow1/Subsystem/If Action Subsystem2 ==
  Action Port : ActionPort  ActionPortLabel=else
  Constant : Constant  Value=0
  Out1 : Outport
  wires:
  Constant/1 -> Out1/1

== system AvionicStateFlow1/Subsystem/If Action Subsystem3 ==
  In1 : Inport
  Action Port : ActionPort  ActionPortLabel=elseif( u1 == 3)
  Out1 : Outport
  wires:
  In1/1 -> Out1/1

== system AvionicStateFlow1/Subsystem/If Action Subsystem4 ==
  In1 : Inport
  Action Port : ActionPort  ActionPortLabel=elseif( u1 == 4)
  Out1 : Outport
  wires:
  In1/1 -> Out1/1

== matlab function AvionicStateFlow1/Kalman filter/MATLAB Function1 ==
  data: Q_d output; R output; Ts output
function [Q_d,R,Ts] = fcn()
Ts = 0.01;

Q_c = 1e-6*diag([1 1 100]);
Q_d = Ts*Q_c;
R = 1e-1*diag([10 5]);

== matlab function AvionicStateFlow1/Global acceleration/MATLAB Function ==
  data: a input; acc output; b input
function acc = fcn(a,b)
b1= b(1)*pi/180; %roll
b2 = b(2)*pi/180; %pitch
b3 = b(3)*pi/180; %yaw
Rz = [cos(b3) sin(b3) 0 ;
    -sin(b3) cos(b3) 0;
    0 0 1];

Rx = [1 0 0;
    0 cos(b1) sin(b1);
    0 -sin(b1) cos(b1)];

Ry = [cos(b2) 0 -sin(b2);
    0 1 0;
    sin(b2) 0 cos(b2)];

acc = (Rx*Ry*Rz)'*a;

== stateflow chart AvionicStateFlow1/Chart ==
  state OnLaunchPad
    y=0;
  state LaunchDetect
    y=1;
  state ApogeeDetect
    y=2;
  state Droping
    y=3;
  state TouchDown
    y=4;
  (default) -> OnLaunchPad
  OnLaunchPad -> LaunchDetect : [a>9.81*3]
  LaunchDetect -> ApogeeDetect : [v<=0.5 & h>20]
  ApogeeDetect -> Droping : after(3,sec)
  Droping -> TouchDown : [abs(a)>5*9.81]
  data: a input; y output; v input; h input

== matlab function AvionicStateFlow1/Kalman filter/MATLAB Function2 ==
  data: Q_d input; R input; hp input; dh input; x output; Ts input; uk input; P_trace output
function [x, P_trace] = fcn(Q_d, R, hp,dh, Ts, uk)
persistent x_est_p P;   
if isempty(x_est_p)
       x_est_p = [0;0;0]; P = eye(3);
end
   A = [0 1 0; 0 0 1; 0 0 0]; 
   B = [Ts/2; 1; 0];
   C = [1 0 0 ; 0 1 0]; 
   
   Ak = eye(3)+A*Ts;
   Bk = B*Ts;
   Ck = C;

   y_est = Ck*x_est_p;
   %Compute kalman gain
   wk = P*Ck'/(Ck*P*Ck'+R); 
   %update predicted value
   x = x_est_p + wk*([hp;dh] - y_est);
   %Compute prediction at the nest time step
   x_est = Ak*x + Bk*uk;
   %Update error covariance matrices
   P = P - wk*Ck*P;
   P = Ak*P*Ak' + Q_d;
   P_trace = trace(P);
   x_est_p =x_est;

== matlab function AvionicStateFlow1/ALTITUDE /MATLAB Function ==
  data: p input; rho output; t input
function rho = fcn(p,t)

M = 0.0289644; %kg/mol\
R = 8.31432; %Nm/molK

rho = (M*p)/(R*t);

== matlab function AvionicStateFlow1/ALTITUDE /MATLAB Function1 ==
  data: rho input; h_AGL output; p input; Pre output
function [h_AGL, Pre]= fcn(rho,p)
P0 = 101325; %N/m^2
g = 9.80665; %m/s^2
hg = 14.3256; %m 
Pre = p-P0;
h = (Pre)/-(rho*g);
h_AGL = h-hg

== matlab function AvionicStateFlow1/GPS/MATLAB Function1 ==
  data: raw_val input; y output
function y = fcn(raw_val)
decimal_val = raw_val/100;
degrees = fix(decimal_val)
mm_mmmm =(decimal_val-fix(decimal_val))/0.6
y = degrees +mm_mmmm;

== matlab function AvionicStateFlow1/GPS/MATLAB Function2 ==
  data: raw_val input; y output
function y = fcn(raw_val)
decimal_val = raw_val/100;
degrees = fix(decimal_val)
mm_mmmm =(decimal_val-fix(decimal_val))/0.6
y = degrees +mm_mmmm;
